simulink model "discretefourierxform"  (R2017a)
settings: Solver=VariableStepAuto  StartTime=0.0  StopTime=10.0  RelTol=1e-3
settings Model: Creator=dangd  LastModifiedBy=dangd

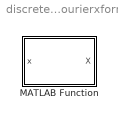
== system discretefourierxform ==
  MATLAB Function : MATLAB Function  TreatAsAtomicUnit=on

== matlab function discretefourierxform/MATLAB Function ==
  data: x input; X output
function X = fcn(x)

i = sqrt(-1);
N = length(x);
w = -pi:0.1:pi;
X = zeros(length(w), 1);

for k = 1:length(w)
    for n = 1:N
        X(k) = X(k) + (x(n) * exp(-i*w(k)*(n+(-4)-1)));
    end
end
